simulink model "neuronchainv3"  (Simulink 7.6)
settings: Solver=ode45  StartTime=0.0  StopTime=10.0  RelTol=1e-3
values from neighbouring files (symbols this model uses):
  alpha = 0.8    [excneuroninit.m]
  beta = 0.05    [excneuroninit.m]
  sigslopef = 1    [excneuroninit.m]
  sigslopei = 3    [excneuroninit.m]
  tau_s = 5    [excneuroninit.m]
libraries: simulink x480, neuronpoolibv3 x3
(part 10 of 17)

== system neuronchainv3/Hebbcon2p2/32/h(ui) ==
  x : Inport
  Constant : Constant  Value=offset
  Constant1 : Constant  Value=slope
  Constant2 : Constant
  Gain : Gain  Gain=-1  SaturateOnIntegerOverflow=on  OutDataTypeStr=Inherit: Same as input  ParamDataTypeStr=Inherit: Same as input
  Math Function : Math  SaturateOnIntegerOverflow=on
  Math Function1 : Math  Operator=reciprocal  SaturateOnIntegerOverflow=on
  Model Info : simulink/Model-Wide Utilities/Model Info  SystemSampleTime=-1  InitialBlockCM=None  BlockCM=None  Frame=on  DisplayStringWithTags=|  HorizontalTextAlignment=Center  LeftAlignmentValue=0.5  SourceBlockDiagram=excneuronv3  TagMaxNumber=20
      | Model Info
      | %<Creator> Han, Cheol
  Product : Product  SaturateOnIntegerOverflow=on  OutDataTypeStr=Inherit: Same as first input
  Sum : Sum  Inputs=+-  SaturateOnIntegerOverflow=on
  Sum1 : Sum  SaturateOnIntegerOverflow=on
  y : Outport  InitialOutput=0
  wires:
  x/1 -> Sum/1
  Constant/1 -> Sum/2
  Sum/1 -> Product/1
  Constant1/1 -> Product/2
  Product/1 -> Gain/1
  Gain/1 -> Math Function/1
  Math Function/1 -> Sum1/1
  Constant2/1 -> Sum1/2
  Sum1/1 -> Math Function1/1
  Math Function1/1 -> y/1

== system neuronchainv3/Hebbcon2p2/33/f(ui) ==
  x : Inport
  Constant : Constant  Value=offset
  Constant1 : Constant  Value=slope
  Constant2 : Constant
  Gain : Gain  Gain=-1  SaturateOnIntegerOverflow=on  OutDataTypeStr=Inherit: Same as input  ParamDataTypeStr=Inherit: Same as input
  Math Function : Math  SaturateOnIntegerOverflow=on
  Math Function1 : Math  Operator=reciprocal  SaturateOnIntegerOverflow=on
  Model Info : simulink/Model-Wide Utilities/Model Info  SystemSampleTime=-1  InitialBlockCM=None  BlockCM=None  Frame=on  DisplayStringWithTags=|  HorizontalTextAlignment=Center  LeftAlignmentValue=0.5  SourceBlockDiagram=excneuronv3  TagMaxNumber=20
      | Model Info
      | %<Creator> Han, Cheol
  Product : Product  SaturateOnIntegerOverflow=on  OutDataTypeStr=Inherit: Same as first input
  Sum : Sum  Inputs=+-  SaturateOnIntegerOverflow=on
  Sum1 : Sum  SaturateOnIntegerOverflow=on
  y : Outport  InitialOutput=0
  wires:
  x/1 -> Sum/1
  Constant/1 -> Sum/2
  Sum/1 -> Product/1
  Constant1/1 -> Product/2
  Product/1 -> Gain/1
  Gain/1 -> Math Function/1
  Math Function/1 -> Sum1/1
  Constant2/1 -> Sum1/2
  Sum1/1 -> Math Function1/1
  Math Function1/1 -> y/1

== system neuronchainv3/Hebbcon2p2/33/f(uj) ==
  x : Inport
  Constant : Constant  Value=offset
  Constant1 : Constant  Value=slope
  Constant2 : Constant
  Gain : Gain  Gain=-1  SaturateOnIntegerOverflow=on  OutDataTypeStr=Inherit: Same as input  ParamDataTypeStr=Inherit: Same as input
  Math Function : Math  SaturateOnIntegerOverflow=on
  Math Function1 : Math  Operator=reciprocal  SaturateOnIntegerOverflow=on
  Model Info : simulink/Model-Wide Utilities/Model Info  SystemSampleTime=-1  InitialBlockCM=None  BlockCM=None  Frame=on  DisplayStringWithTags=|  HorizontalTextAlignment=Center  LeftAlignmentValue=0.5  SourceBlockDiagram=excneuronv3  TagMaxNumber=20
      | Model Info
      | %<Creator> Han, Cheol
  Product : Product  SaturateOnIntegerOverflow=on  OutDataTypeStr=Inherit: Same as first input
  Sum : Sum  Inputs=+-  SaturateOnIntegerOverflow=on
  Sum1 : Sum  SaturateOnIntegerOverflow=on
  y : Outport  InitialOutput=0
  wires:
  x/1 -> Sum/1
  Constant/1 -> Sum/2
  Sum/1 -> Product/1
  Constant1/1 -> Product/2
  Product/1 -> Gain/1
  Gain/1 -> Math Function/1
  Math Function/1 -> Sum1/1
  Constant2/1 -> Sum1/2
  Sum1/1 -> Math Function1/1
  Math Function1/1 -> y/1

== system neuronchainv3/Hebbcon2p2/33/h(ui) ==
  x : Inport
  Constant : Constant  Value=offset
  Constant1 : Constant  Value=slope
  Constant2 : Constant
  Gain : Gain  Gain=-1  SaturateOnIntegerOverflow=on  OutDataTypeStr=Inherit: Same as input  ParamDataTypeStr=Inherit: Same as input
  Math Function : Math  SaturateOnIntegerOverflow=on
  Math Function1 : Math  Operator=reciprocal  SaturateOnIntegerOverflow=on
  Model Info : simulink/Model-Wide Utilities/Model Info  SystemSampleTime=-1  InitialBlockCM=None  BlockCM=None  Frame=on  DisplayStringWithTags=|  HorizontalTextAlignment=Center  LeftAlignmentValue=0.5  SourceBlockDiagram=excneuronv3  TagMaxNumber=20
      | Model Info
      | %<Creator> Han, Cheol
  Product : Product  SaturateOnIntegerOverflow=on  OutDataTypeStr=Inherit: Same as first input
  Sum : Sum  Inputs=+-  SaturateOnIntegerOverflow=on
  Sum1 : Sum  SaturateOnIntegerOverflow=on
  y : Outport  InitialOutput=0
  wires:
  x/1 -> Sum/1
  Constant/1 -> Sum/2
  Sum/1 -> Product/1
  Constant1/1 -> Product/2
  Product/1 -> Gain/1
  Gain/1 -> Math Function/1
  Math Function/1 -> Sum1/1
  Constant2/1 -> Sum1/2
  Sum1/1 -> Math Function1/1
  Math Function1/1 -> y/1

== system neuronchainv3/Hebbcon2p2/34/f(ui) ==
  x : Inport
  Constant : Constant  Value=offset
  Constant1 : Constant  Value=slope
  Constant2 : Constant
  Gain : Gain  Gain=-1  SaturateOnIntegerOverflow=on  OutDataTypeStr=Inherit: Same as input  ParamDataTypeStr=Inherit: Same as input
  Math Function : Math  SaturateOnIntegerOverflow=on
  Math Function1 : Math  Operator=reciprocal  SaturateOnIntegerOverflow=on
  Model Info : simulink/Model-Wide Utilities/Model Info  SystemSampleTime=-1  InitialBlockCM=None  BlockCM=None  Frame=on  DisplayStringWithTags=|  HorizontalTextAlignment=Center  LeftAlignmentValue=0.5  SourceBlockDiagram=excneuronv3  TagMaxNumber=20
      | Model Info
      | %<Creator> Han, Cheol
  Product : Product  SaturateOnIntegerOverflow=on  OutDataTypeStr=Inherit: Same as first input
  Sum : Sum  Inputs=+-  SaturateOnIntegerOverflow=on
  Sum1 : Sum  SaturateOnIntegerOverflow=on
  y : Outport  InitialOutput=0
  wires:
  x/1 -> Sum/1
  Constant/1 -> Sum/2
  Sum/1 -> Product/1
  Constant1/1 -> Product/2
  Product/1 -> Gain/1
  Gain/1 -> Math Function/1
  Math Function/1 -> Sum1/1
  Constant2/1 -> Sum1/2
  Sum1/1 -> Math Function1/1
  Math Function1/1 -> y/1

== system neuronchainv3/Hebbcon2p2/34/f(uj) ==
  x : Inport
  Constant : Constant  Value=offset
  Constant1 : Constant  Value=slope
  Constant2 : Constant
  Gain : Gain  Gain=-1  SaturateOnIntegerOverflow=on  OutDataTypeStr=Inherit: Same as input  ParamDataTypeStr=Inherit: Same as input
  Math Function : Math  SaturateOnIntegerOverflow=on
  Math Function1 : Math  Operator=reciprocal  SaturateOnIntegerOverflow=on
  Model Info : simulink/Model-Wide Utilities/Model Info  SystemSampleTime=-1  InitialBlockCM=None  BlockCM=None  Frame=on  DisplayStringWithTags=|  HorizontalTextAlignment=Center  LeftAlignmentValue=0.5  SourceBlockDiagram=excneuronv3  TagMaxNumber=20
      | Model Info
      | %<Creator> Han, Cheol
  Product : Product  SaturateOnIntegerOverflow=on  OutDataTypeStr=Inherit: Same as first input
  Sum : Sum  Inputs=+-  SaturateOnIntegerOverflow=on
  Sum1 : Sum  SaturateOnIntegerOverflow=on
  y : Outport  InitialOutput=0
  wires:
  x/1 -> Sum/1
  Constant/1 -> Sum/2
  Sum/1 -> Product/1
  Constant1/1 -> Product/2
  Product/1 -> Gain/1
  Gain/1 -> Math Function/1
  Math Function/1 -> Sum1/1
  Constant2/1 -> Sum1/2
  Sum1/1 -> Math Function1/1
  Math Function1/1 -> y/1

== system neuronchainv3/Hebbcon2p2/34/h(ui) ==
  x : Inport
  Constant : Constant  Value=offset
  Constant1 : Constant  Value=slope
  Constant2 : Constant
  Gain : Gain  Gain=-1  SaturateOnIntegerOverflow=on  OutDataTypeStr=Inherit: Same as input  ParamDataTypeStr=Inherit: Same as input
  Math Function : Math  SaturateOnIntegerOverflow=on
  Math Function1 : Math  Operator=reciprocal  SaturateOnIntegerOverflow=on
  Model Info : simulink/Model-Wide Utilities/Model Info  SystemSampleTime=-1  InitialBlockCM=None  BlockCM=None  Frame=on  DisplayStringWithTags=|  HorizontalTextAlignment=Center  LeftAlignmentValue=0.5  SourceBlockDiagram=excneuronv3  TagMaxNumber=20
      | Model Info
      | %<Creator> Han, Cheol
  Product : Product  SaturateOnIntegerOverflow=on  OutDataTypeStr=Inherit: Same as first input
  Sum : Sum  Inputs=+-  SaturateOnIntegerOverflow=on
  Sum1 : Sum  SaturateOnIntegerOverflow=on
  y : Outport  InitialOutput=0
  wires:
  x/1 -> Sum/1
  Constant/1 -> Sum/2
  Sum/1 -> Product/1
  Constant1/1 -> Product/2
  Product/1 -> Gain/1
  Gain/1 -> Math Function/1
  Math Function/1 -> Sum1/1
  Constant2/1 -> Sum1/2
  Sum1/1 -> Math Function1/1
  Math Function1/1 -> y/1

== system neuronchainv3/Hebbcon2p2/35/f(ui) ==
  x : Inport
  Constant : Constant  Value=offset
  Constant1 : Constant  Value=slope
  Constant2 : Constant
  Gain : Gain  Gain=-1  SaturateOnIntegerOverflow=on  OutDataTypeStr=Inherit: Same as input  ParamDataTypeStr=Inherit: Same as input
  Math Function : Math  SaturateOnIntegerOverflow=on
  Math Function1 : Math  Operator=reciprocal  SaturateOnIntegerOverflow=on
  Model Info : simulink/Model-Wide Utilities/Model Info  SystemSampleTime=-1  InitialBlockCM=None  BlockCM=None  Frame=on  DisplayStringWithTags=|  HorizontalTextAlignment=Center  LeftAlignmentValue=0.5  SourceBlockDiagram=excneuronv3  TagMaxNumber=20
      | Model Info
      | %<Creator> Han, Cheol
  Product : Product  SaturateOnIntegerOverflow=on  OutDataTypeStr=Inherit: Same as first input
  Sum : Sum  Inputs=+-  SaturateOnIntegerOverflow=on
  Sum1 : Sum  SaturateOnIntegerOverflow=on
  y : Outport  InitialOutput=0
  wires:
  x/1 -> Sum/1
  Constant/1 -> Sum/2
  Sum/1 -> Product/1
  Constant1/1 -> Product/2
  Product/1 -> Gain/1
  Gain/1 -> Math Function/1
  Math Function/1 -> Sum1/1
  Constant2/1 -> Sum1/2
  Sum1/1 -> Math Function1/1
  Math Function1/1 -> y/1

== system neuronchainv3/Hebbcon2p2/35/f(uj) ==
  x : Inport
  Constant : Constant  Value=offset
  Constant1 : Constant  Value=slope
  Constant2 : Constant
  Gain : Gain  Gain=-1  SaturateOnIntegerOverflow=on  OutDataTypeStr=Inherit: Same as input  ParamDataTypeStr=Inherit: Same as input
  Math Function : Math  SaturateOnIntegerOverflow=on
  Math Function1 : Math  Operator=reciprocal  SaturateOnIntegerOverflow=on
  Model Info : simulink/Model-Wide Utilities/Model Info  SystemSampleTime=-1  InitialBlockCM=None  BlockCM=None  Frame=on  DisplayStringWithTags=|  HorizontalTextAlignment=Center  LeftAlignmentValue=0.5  SourceBlockDiagram=excneuronv3  TagMaxNumber=20
      | Model Info
      | %<Creator> Han, Cheol
  Product : Product  SaturateOnIntegerOverflow=on  OutDataTypeStr=Inherit: Same as first input
  Sum : Sum  Inputs=+-  SaturateOnIntegerOverflow=on
  Sum1 : Sum  SaturateOnIntegerOverflow=on
  y : Outport  InitialOutput=0
  wires:
  x/1 -> Sum/1
  Constant/1 -> Sum/2
  Sum/1 -> Product/1
  Constant1/1 -> Product/2
  Product/1 -> Gain/1
  Gain/1 -> Math Function/1
  Math Function/1 -> Sum1/1
  Constant2/1 -> Sum1/2
  Sum1/1 -> Math Function1/1
  Math Function1/1 -> y/1

== system neuronchainv3/Hebbcon2p2/35/h(ui) ==
  x : Inport
  Constant : Constant  Value=offset
  Constant1 : Constant  Value=slope
  Constant2 : Constant
  Gain : Gain  Gain=-1  SaturateOnIntegerOverflow=on  OutDataTypeStr=Inherit: Same as input  ParamDataTypeStr=Inherit: Same as input
  Math Function : Math  SaturateOnIntegerOverflow=on
  Math Function1 : Math  Operator=reciprocal  SaturateOnIntegerOverflow=on
  Model Info : simulink/Model-Wide Utilities/Model Info  SystemSampleTime=-1  InitialBlockCM=None  BlockCM=None  Frame=on  DisplayStringWithTags=|  HorizontalTextAlignment=Center  LeftAlignmentValue=0.5  SourceBlockDiagram=excneuronv3  TagMaxNumber=20
      | Model Info
      | %<Creator> Han, Cheol
  Product : Product  SaturateOnIntegerOverflow=on  OutDataTypeStr=Inherit: Same as first input
  Sum : Sum  Inputs=+-  SaturateOnIntegerOverflow=on
  Sum1 : Sum  SaturateOnIntegerOverflow=on
  y : Outport  InitialOutput=0
  wires:
  x/1 -> Sum/1
  Constant/1 -> Sum/2
  Sum/1 -> Product/1
  Constant1/1 -> Product/2
  Product/1 -> Gain/1
  Gain/1 -> Math Function/1
  Math Function/1 -> Sum1/1
  Constant2/1 -> Sum1/2
  Sum1/1 -> Math Function1/1
  Math Function1/1 -> y/1

== system neuronchainv3/Hebbcon2p2/4/f(ui) ==
  x : Inport
  Constant : Constant  Value=offset
  Constant1 : Constant  Value=slope
  Constant2 : Constant
  Gain : Gain  Gain=-1  SaturateOnIntegerOverflow=on  OutDataTypeStr=Inherit: Same as input  ParamDataTypeStr=Inherit: Same as input
  Math Function : Math  SaturateOnIntegerOverflow=on
  Math Function1 : Math  Operator=reciprocal  SaturateOnIntegerOverflow=on
  Model Info : simulink/Model-Wide Utilities/Model Info  SystemSampleTime=-1  InitialBlockCM=None  BlockCM=None  Frame=on  DisplayStringWithTags=|  HorizontalTextAlignment=Center  LeftAlignmentValue=0.5  SourceBlockDiagram=excneuronv3  TagMaxNumber=20
      | Model Info
      | %<Creator> Han, Cheol
  Product : Product  SaturateOnIntegerOverflow=on  OutDataTypeStr=Inherit: Same as first input
  Sum : Sum  Inputs=+-  SaturateOnIntegerOverflow=on
  Sum1 : Sum  SaturateOnIntegerOverflow=on
  y : Outport  InitialOutput=0
  wires:
  x/1 -> Sum/1
  Constant/1 -> Sum/2
  Sum/1 -> Product/1
  Constant1/1 -> Product/2
  Product/1 -> Gain/1
  Gain/1 -> Math Function/1
  Math Function/1 -> Sum1/1
  Constant2/1 -> Sum1/2
  Sum1/1 -> Math Function1/1
  Math Function1/1 -> y/1

== system neuronchainv3/Hebbcon2p2/4/f(uj) ==
  x : Inport
  Constant : Constant  Value=offset
  Constant1 : Constant  Value=slope
  Constant2 : Constant
  Gain : Gain  Gain=-1  SaturateOnIntegerOverflow=on  OutDataTypeStr=Inherit: Same as input  ParamDataTypeStr=Inherit: Same as input
  Math Function : Math  SaturateOnIntegerOverflow=on
  Math Function1 : Math  Operator=reciprocal  SaturateOnIntegerOverflow=on
  Model Info : simulink/Model-Wide Utilities/Model Info  SystemSampleTime=-1  InitialBlockCM=None  BlockCM=None  Frame=on  DisplayStringWithTags=|  HorizontalTextAlignment=Center  LeftAlignmentValue=0.5  SourceBlockDiagram=excneuronv3  TagMaxNumber=20
      | Model Info
      | %<Creator> Han, Cheol
  Product : Product  SaturateOnIntegerOverflow=on  OutDataTypeStr=Inherit: Same as first input
  Sum : Sum  Inputs=+-  SaturateOnIntegerOverflow=on
  Sum1 : Sum  SaturateOnIntegerOverflow=on
  y : Outport  InitialOutput=0
  wires:
  x/1 -> Sum/1
  Constant/1 -> Sum/2
  Sum/1 -> Product/1
  Constant1/1 -> Product/2
  Product/1 -> Gain/1
  Gain/1 -> Math Function/1
  Math Function/1 -> Sum1/1
  Constant2/1 -> Sum1/2
  Sum1/1 -> Math Function1/1
  Math Function1/1 -> y/1

== system neuronchainv3/Hebbcon2p2/4/h(ui) ==
  x : Inport
  Constant : Constant  Value=offset
  Constant1 : Constant  Value=slope
  Constant2 : Constant
  Gain : Gain  Gain=-1  SaturateOnIntegerOverflow=on  OutDataTypeStr=Inherit: Same as input  ParamDataTypeStr=Inherit: Same as input
  Math Function : Math  SaturateOnIntegerOverflow=on
  Math Function1 : Math  Operator=reciprocal  SaturateOnIntegerOverflow=on
  Model Info : simulink/Model-Wide Utilities/Model Info  SystemSampleTime=-1  InitialBlockCM=None  BlockCM=None  Frame=on  DisplayStringWithTags=|  HorizontalTextAlignment=Center  LeftAlignmentValue=0.5  SourceBlockDiagram=excneuronv3  TagMaxNumber=20
      | Model Info
      | %<Creator> Han, Cheol
  Product : Product  SaturateOnIntegerOverflow=on  OutDataTypeStr=Inherit: Same as first input
  Sum : Sum  Inputs=+-  SaturateOnIntegerOverflow=on
  Sum1 : Sum  SaturateOnIntegerOverflow=on
  y : Outport  InitialOutput=0
  wires:
  x/1 -> Sum/1
  Constant/1 -> Sum/2
  Sum/1 -> Product/1
  Constant1/1 -> Product/2
  Product/1 -> Gain/1
  Gain/1 -> Math Function/1
  Math Function/1 -> Sum1/1
  Constant2/1 -> Sum1/2
  Sum1/1 -> Math Function1/1
  Math Function1/1 -> y/1

== system neuronchainv3/Hebbcon2p2/41/f(ui) ==
  x : Inport
  Constant : Constant  Value=offset
  Constant1 : Constant  Value=slope
  Constant2 : Constant
  Gain : Gain  Gain=-1  SaturateOnIntegerOverflow=on  OutDataTypeStr=Inherit: Same as input  ParamDataTypeStr=Inherit: Same as input
  Math Function : Math  SaturateOnIntegerOverflow=on
  Math Function1 : Math  Operator=reciprocal  SaturateOnIntegerOverflow=on
  Model Info : simulink/Model-Wide Utilities/Model Info  SystemSampleTime=-1  InitialBlockCM=None  BlockCM=None  Frame=on  DisplayStringWithTags=|  HorizontalTextAlignment=Center  LeftAlignmentValue=0.5  SourceBlockDiagram=excneuronv3  TagMaxNumber=20
      | Model Info
      | %<Creator> Han, Cheol
  Product : Product  SaturateOnIntegerOverflow=on  OutDataTypeStr=Inherit: Same as first input
  Sum : Sum  Inputs=+-  SaturateOnIntegerOverflow=on
  Sum1 : Sum  SaturateOnIntegerOverflow=on
  y : Outport  InitialOutput=0
  wires:
  x/1 -> Sum/1
  Constant/1 -> Sum/2
  Sum/1 -> Product/1
  Constant1/1 -> Product/2
  Product/1 -> Gain/1
  Gain/1 -> Math Function/1
  Math Function/1 -> Sum1/1
  Constant2/1 -> Sum1/2
  Sum1/1 -> Math Function1/1
  Math Function1/1 -> y/1

== system neuronchainv3/Hebbcon2p2/41/f(uj) ==
  x : Inport
  Constant : Constant  Value=offset
  Constant1 : Constant  Value=slope
  Constant2 : Constant
  Gain : Gain  Gain=-1  SaturateOnIntegerOverflow=on  OutDataTypeStr=Inherit: Same as input  ParamDataTypeStr=Inherit: Same as input
  Math Function : Math  SaturateOnIntegerOverflow=on
  Math Function1 : Math  Operator=reciprocal  SaturateOnIntegerOverflow=on
  Model Info : simulink/Model-Wide Utilities/Model Info  SystemSampleTime=-1  InitialBlockCM=None  BlockCM=None  Frame=on  DisplayStringWithTags=|  HorizontalTextAlignment=Center  LeftAlignmentValue=0.5  SourceBlockDiagram=excneuronv3  TagMaxNumber=20
      | Model Info
      | %<Creator> Han, Cheol
  Product : Product  SaturateOnIntegerOverflow=on  OutDataTypeStr=Inherit: Same as first input
  Sum : Sum  Inputs=+-  SaturateOnIntegerOverflow=on
  Sum1 : Sum  SaturateOnIntegerOverflow=on
  y : Outport  InitialOutput=0
  wires:
  x/1 -> Sum/1
  Constant/1 -> Sum/2
  Sum/1 -> Product/1
  Constant1/1 -> Product/2
  Product/1 -> Gain/1
  Gain/1 -> Math Function/1
  Math Function/1 -> Sum1/1
  Constant2/1 -> Sum1/2
  Sum1/1 -> Math Function1/1
  Math Function1/1 -> y/1

== system neuronchainv3/Hebbcon2p2/41/h(ui) ==
  x : Inport
  Constant : Constant  Value=offset
  Constant1 : Constant  Value=slope
  Constant2 : Constant
  Gain : Gain  Gain=-1  SaturateOnIntegerOverflow=on  OutDataTypeStr=Inherit: Same as input  ParamDataTypeStr=Inherit: Same as input
  Math Function : Math  SaturateOnIntegerOverflow=on
  Math Function1 : Math  Operator=reciprocal  SaturateOnIntegerOverflow=on
  Model Info : simulink/Model-Wide Utilities/Model Info  SystemSampleTime=-1  InitialBlockCM=None  BlockCM=None  Frame=on  DisplayStringWithTags=|  HorizontalTextAlignment=Center  LeftAlignmentValue=0.5  SourceBlockDiagram=excneuronv3  TagMaxNumber=20
      | Model Info
      | %<Creator> Han, Cheol
  Product : Product  SaturateOnIntegerOverflow=on  OutDataTypeStr=Inherit: Same as first input
  Sum : Sum  Inputs=+-  SaturateOnIntegerOverflow=on
  Sum1 : Sum  SaturateOnIntegerOverflow=on
  y : Outport  InitialOutput=0
  wires:
  x/1 -> Sum/1
  Constant/1 -> Sum/2
  Sum/1 -> Product/1
  Constant1/1 -> Product/2
  Product/1 -> Gain/1
  Gain/1 -> Math Function/1
  Math Function/1 -> Sum1/1
  Constant2/1 -> Sum1/2
  Sum1/1 -> Math Function1/1
  Math Function1/1 -> y/1

== system neuronchainv3/Hebbcon2p2/42/f(ui) ==
  x : Inport
  Constant : Constant  Value=offset
  Constant1 : Constant  Value=slope
  Constant2 : Constant
  Gain : Gain  Gain=-1  SaturateOnIntegerOverflow=on  OutDataTypeStr=Inherit: Same as input  ParamDataTypeStr=Inherit: Same as input
  Math Function : Math  SaturateOnIntegerOverflow=on
  Math Function1 : Math  Operator=reciprocal  SaturateOnIntegerOverflow=on
  Model Info : simulink/Model-Wide Utilities/Model Info  SystemSampleTime=-1  InitialBlockCM=None  BlockCM=None  Frame=on  DisplayStringWithTags=|  HorizontalTextAlignment=Center  LeftAlignmentValue=0.5  SourceBlockDiagram=excneuronv3  TagMaxNumber=20
      | Model Info
      | %<Creator> Han, Cheol
  Product : Product  SaturateOnIntegerOverflow=on  OutDataTypeStr=Inherit: Same as first input
  Sum : Sum  Inputs=+-  SaturateOnIntegerOverflow=on
  Sum1 : Sum  SaturateOnIntegerOverflow=on
  y : Outport  InitialOutput=0
  wires:
  x/1 -> Sum/1
  Constant/1 -> Sum/2
  Sum/1 -> Product/1
  Constant1/1 -> Product/2
  Product/1 -> Gain/1
  Gain/1 -> Math Function/1
  Math Function/1 -> Sum1/1
  Constant2/1 -> Sum1/2
  Sum1/1 -> Math Function1/1
  Math Function1/1 -> y/1

== system neuronchainv3/Hebbcon2p2/42/f(uj) ==
  x : Inport
  Constant : Constant  Value=offset
  Constant1 : Constant  Value=slope
  Constant2 : Constant
  Gain : Gain  Gain=-1  SaturateOnIntegerOverflow=on  OutDataTypeStr=Inherit: Same as input  ParamDataTypeStr=Inherit: Same as input
  Math Function : Math  SaturateOnIntegerOverflow=on
  Math Function1 : Math  Operator=reciprocal  SaturateOnIntegerOverflow=on
  Model Info : simulink/Model-Wide Utilities/Model Info  SystemSampleTime=-1  InitialBlockCM=None  BlockCM=None  Frame=on  DisplayStringWithTags=|  HorizontalTextAlignment=Center  LeftAlignmentValue=0.5  SourceBlockDiagram=excneuronv3  TagMaxNumber=20
      | Model Info
      | %<Creator> Han, Cheol
  Product : Product  SaturateOnIntegerOverflow=on  OutDataTypeStr=Inherit: Same as first input
  Sum : Sum  Inputs=+-  SaturateOnIntegerOverflow=on
  Sum1 : Sum  SaturateOnIntegerOverflow=on
  y : Outport  InitialOutput=0
  wires:
  x/1 -> Sum/1
  Constant/1 -> Sum/2
  Sum/1 -> Product/1
  Constant1/1 -> Product/2
  Product/1 -> Gain/1
  Gain/1 -> Math Function/1
  Math Function/1 -> Sum1/1
  Constant2/1 -> Sum1/2
  Sum1/1 -> Math Function1/1
  Math Function1/1 -> y/1

== system neuronchainv3/Hebbcon2p2/42/h(ui) ==
  x : Inport
  Constant : Constant  Value=offset
  Constant1 : Constant  Value=slope
  Constant2 : Constant
  Gain : Gain  Gain=-1  SaturateOnIntegerOverflow=on  OutDataTypeStr=Inherit: Same as input  ParamDataTypeStr=Inherit: Same as input
  Math Function : Math  SaturateOnIntegerOverflow=on
  Math Function1 : Math  Operator=reciprocal  SaturateOnIntegerOverflow=on
  Model Info : simulink/Model-Wide Utilities/Model Info  SystemSampleTime=-1  InitialBlockCM=None  BlockCM=None  Frame=on  DisplayStringWithTags=|  HorizontalTextAlignment=Center  LeftAlignmentValue=0.5  SourceBlockDiagram=excneuronv3  TagMaxNumber=20
      | Model Info
      | %<Creator> Han, Cheol
  Product : Product  SaturateOnIntegerOverflow=on  OutDataTypeStr=Inherit: Same as first input
  Sum : Sum  Inputs=+-  SaturateOnIntegerOverflow=on
  Sum1 : Sum  SaturateOnIntegerOverflow=on
  y : Outport  InitialOutput=0
  wires:
  x/1 -> Sum/1
  Constant/1 -> Sum/2
  Sum/1 -> Product/1
  Constant1/1 -> Product/2
  Product/1 -> Gain/1
  Gain/1 -> Math Function/1
  Math Function/1 -> Sum1/1
  Constant2/1 -> Sum1/2
  Sum1/1 -> Math Function1/1
  Math Function1/1 -> y/1

== system neuronchainv3/Hebbcon2p2/43/f(ui) ==
  x : Inport
  Constant : Constant  Value=offset
  Constant1 : Constant  Value=slope
  Constant2 : Constant
  Gain : Gain  Gain=-1  SaturateOnIntegerOverflow=on  OutDataTypeStr=Inherit: Same as input  ParamDataTypeStr=Inherit: Same as input
  Math Function : Math  SaturateOnIntegerOverflow=on
  Math Function1 : Math  Operator=reciprocal  SaturateOnIntegerOverflow=on
  Model Info : simulink/Model-Wide Utilities/Model Info  SystemSampleTime=-1  InitialBlockCM=None  BlockCM=None  Frame=on  DisplayStringWithTags=|  HorizontalTextAlignment=Center  LeftAlignmentValue=0.5  SourceBlockDiagram=excneuronv3  TagMaxNumber=20
      | Model Info
      | %<Creator> Han, Cheol
  Product : Product  SaturateOnIntegerOverflow=on  OutDataTypeStr=Inherit: Same as first input
  Sum : Sum  Inputs=+-  SaturateOnIntegerOverflow=on
  Sum1 : Sum  SaturateOnIntegerOverflow=on
  y : Outport  InitialOutput=0
  wires:
  x/1 -> Sum/1
  Constant/1 -> Sum/2
  Sum/1 -> Product/1
  Constant1/1 -> Product/2
  Product/1 -> Gain/1
  Gain/1 -> Math Function/1
  Math Function/1 -> Sum1/1
  Constant2/1 -> Sum1/2
  Sum1/1 -> Math Function1/1
  Math Function1/1 -> y/1

== system neuronchainv3/Hebbcon2p2/43/f(uj) ==
  x : Inport
  Constant : Constant  Value=offset
  Constant1 : Constant  Value=slope
  Constant2 : Constant
  Gain : Gain  Gain=-1  SaturateOnIntegerOverflow=on  OutDataTypeStr=Inherit: Same as input  ParamDataTypeStr=Inherit: Same as input
  Math Function : Math  SaturateOnIntegerOverflow=on
  Math Function1 : Math  Operator=reciprocal  SaturateOnIntegerOverflow=on
  Model Info : simulink/Model-Wide Utilities/Model Info  SystemSampleTime=-1  InitialBlockCM=None  BlockCM=None  Frame=on  DisplayStringWithTags=|  HorizontalTextAlignment=Center  LeftAlignmentValue=0.5  SourceBlockDiagram=excneuronv3  TagMaxNumber=20
      | Model Info
      | %<Creator> Han, Cheol
  Product : Product  SaturateOnIntegerOverflow=on  OutDataTypeStr=Inherit: Same as first input
  Sum : Sum  Inputs=+-  SaturateOnIntegerOverflow=on
  Sum1 : Sum  SaturateOnIntegerOverflow=on
  y : Outport  InitialOutput=0
  wires:
  x/1 -> Sum/1
  Constant/1 -> Sum/2
  Sum/1 -> Product/1
  Constant1/1 -> Product/2
  Product/1 -> Gain/1
  Gain/1 -> Math Function/1
  Math Function/1 -> Sum1/1
  Constant2/1 -> Sum1/2
  Sum1/1 -> Math Function1/1
  Math Function1/1 -> y/1

== system neuronchainv3/Hebbcon2p2/43/h(ui) ==
  x : Inport
  Constant : Constant  Value=offset
  Constant1 : Constant  Value=slope
  Constant2 : Constant
  Gain : Gain  Gain=-1  SaturateOnIntegerOverflow=on  OutDataTypeStr=Inherit: Same as input  ParamDataTypeStr=Inherit: Same as input
  Math Function : Math  SaturateOnIntegerOverflow=on
  Math Function1 : Math  Operator=reciprocal  SaturateOnIntegerOverflow=on
  Model Info : simulink/Model-Wide Utilities/Model Info  SystemSampleTime=-1  InitialBlockCM=None  BlockCM=None  Frame=on  DisplayStringWithTags=|  HorizontalTextAlignment=Center  LeftAlignmentValue=0.5  SourceBlockDiagram=excneuronv3  TagMaxNumber=20
      | Model Info
      | %<Creator> Han, Cheol
  Product : Product  SaturateOnIntegerOverflow=on  OutDataTypeStr=Inherit: Same as first input
  Sum : Sum  Inputs=+-  SaturateOnIntegerOverflow=on
  Sum1 : Sum  SaturateOnIntegerOverflow=on
  y : Outport  InitialOutput=0
  wires:
  x/1 -> Sum/1
  Constant/1 -> Sum/2
  Sum/1 -> Product/1
  Constant1/1 -> Product/2
  Product/1 -> Gain/1
  Gain/1 -> Math Function/1
  Math Function/1 -> Sum1/1
  Constant2/1 -> Sum1/2
  Sum1/1 -> Math Function1/1
  Math Function1/1 -> y/1

== system neuronchainv3/Hebbcon2p2/44/f(ui) ==
  x : Inport
  Constant : Constant  Value=offset
  Constant1 : Constant  Value=slope
  Constant2 : Constant
  Gain : Gain  Gain=-1  SaturateOnIntegerOverflow=on  OutDataTypeStr=Inherit: Same as input  ParamDataTypeStr=Inherit: Same as input
  Math Function : Math  SaturateOnIntegerOverflow=on
  Math Function1 : Math  Operator=reciprocal  SaturateOnIntegerOverflow=on
  Model Info : simulink/Model-Wide Utilities/Model Info  SystemSampleTime=-1  InitialBlockCM=None  BlockCM=None  Frame=on  DisplayStringWithTags=|  HorizontalTextAlignment=Center  LeftAlignmentValue=0.5  SourceBlockDiagram=excneuronv3  TagMaxNumber=20
      | Model Info
      | %<Creator> Han, Cheol
  Product : Product  SaturateOnIntegerOverflow=on  OutDataTypeStr=Inherit: Same as first input
  Sum : Sum  Inputs=+-  SaturateOnIntegerOverflow=on
  Sum1 : Sum  SaturateOnIntegerOverflow=on
  y : Outport  InitialOutput=0
  wires:
  x/1 -> Sum/1
  Constant/1 -> Sum/2
  Sum/1 -> Product/1
  Constant1/1 -> Product/2
  Product/1 -> Gain/1
  Gain/1 -> Math Function/1
  Math Function/1 -> Sum1/1
  Constant2/1 -> Sum1/2
  Sum1/1 -> Math Function1/1
  Math Function1/1 -> y/1

== system neuronchainv3/Hebbcon2p2/44/f(uj) ==
  x : Inport
  Constant : Constant  Value=offset
  Constant1 : Constant  Value=slope
  Constant2 : Constant
  Gain : Gain  Gain=-1  SaturateOnIntegerOverflow=on  OutDataTypeStr=Inherit: Same as input  ParamDataTypeStr=Inherit: Same as input
  Math Function : Math  SaturateOnIntegerOverflow=on
  Math Function1 : Math  Operator=reciprocal  SaturateOnIntegerOverflow=on
  Model Info : simulink/Model-Wide Utilities/Model Info  SystemSampleTime=-1  InitialBlockCM=None  BlockCM=None  Frame=on  DisplayStringWithTags=|  HorizontalTextAlignment=Center  LeftAlignmentValue=0.5  SourceBlockDiagram=excneuronv3  TagMaxNumber=20
      | Model Info
      | %<Creator> Han, Cheol
  Product : Product  SaturateOnIntegerOverflow=on  OutDataTypeStr=Inherit: Same as first input
  Sum : Sum  Inputs=+-  SaturateOnIntegerOverflow=on
  Sum1 : Sum  SaturateOnIntegerOverflow=on
  y : Outport  InitialOutput=0
  wires:
  x/1 -> Sum/1
  Constant/1 -> Sum/2
  Sum/1 -> Product/1
  Constant1/1 -> Product/2
  Product/1 -> Gain/1
  Gain/1 -> Math Function/1
  Math Function/1 -> Sum1/1
  Constant2/1 -> Sum1/2
  Sum1/1 -> Math Function1/1
  Math Function1/1 -> y/1

== system neuronchainv3/Hebbcon2p2/44/h(ui) ==
  x : Inport
  Constant : Constant  Value=offset
  Constant1 : Constant  Value=slope
  Constant2 : Constant
  Gain : Gain  Gain=-1  SaturateOnIntegerOverflow=on  OutDataTypeStr=Inherit: Same as input  ParamDataTypeStr=Inherit: Same as input
  Math Function : Math  SaturateOnIntegerOverflow=on
  Math Function1 : Math  Operator=reciprocal  SaturateOnIntegerOverflow=on
  Model Info : simulink/Model-Wide Utilities/Model Info  SystemSampleTime=-1  InitialBlockCM=None  BlockCM=None  Frame=on  DisplayStringWithTags=|  HorizontalTextAlignment=Center  LeftAlignmentValue=0.5  SourceBlockDiagram=excneuronv3  TagMaxNumber=20
      | Model Info
      | %<Creator> Han, Cheol
  Product : Product  SaturateOnIntegerOverflow=on  OutDataTypeStr=Inherit: Same as first input
  Sum : Sum  Inputs=+-  SaturateOnIntegerOverflow=on
  Sum1 : Sum  SaturateOnIntegerOverflow=on
  y : Outport  InitialOutput=0
  wires:
  x/1 -> Sum/1
  Constant/1 -> Sum/2
  Sum/1 -> Product/1
  Constant1/1 -> Product/2
  Product/1 -> Gain/1
  Gain/1 -> Math Function/1
  Math Function/1 -> Sum1/1
  Constant2/1 -> Sum1/2
  Sum1/1 -> Math Function1/1
  Math Function1/1 -> y/1

== system neuronchainv3/Hebbcon2p2/45/f(ui) ==
  x : Inport
  Constant : Constant  Value=offset
  Constant1 : Constant  Value=slope
  Constant2 : Constant
  Gain : Gain  Gain=-1  SaturateOnIntegerOverflow=on  OutDataTypeStr=Inherit: Same as input  ParamDataTypeStr=Inherit: Same as input
  Math Function : Math  SaturateOnIntegerOverflow=on
  Math Function1 : Math  Operator=reciprocal  SaturateOnIntegerOverflow=on
  Model Info : simulink/Model-Wide Utilities/Model Info  SystemSampleTime=-1  InitialBlockCM=None  BlockCM=None  Frame=on  DisplayStringWithTags=|  HorizontalTextAlignment=Center  LeftAlignmentValue=0.5  SourceBlockDiagram=excneuronv3  TagMaxNumber=20
      | Model Info
      | %<Creator> Han, Cheol
  Product : Product  SaturateOnIntegerOverflow=on  OutDataTypeStr=Inherit: Same as first input
  Sum : Sum  Inputs=+-  SaturateOnIntegerOverflow=on
  Sum1 : Sum  SaturateOnIntegerOverflow=on
  y : Outport  InitialOutput=0
  wires:
  x/1 -> Sum/1
  Constant/1 -> Sum/2
  Sum/1 -> Product/1
  Constant1/1 -> Product/2
  Product/1 -> Gain/1
  Gain/1 -> Math Function/1
  Math Function/1 -> Sum1/1
  Constant2/1 -> Sum1/2
  Sum1/1 -> Math Function1/1
  Math Function1/1 -> y/1

== system neuronchainv3/Hebbcon2p2/45/f(uj) ==
  x : Inport
  Constant : Constant  Value=offset
  Constant1 : Constant  Value=slope
  Constant2 : Constant
  Gain : Gain  Gain=-1  SaturateOnIntegerOverflow=on  OutDataTypeStr=Inherit: Same as input  ParamDataTypeStr=Inherit: Same as input
  Math Function : Math  SaturateOnIntegerOverflow=on
  Math Function1 : Math  Operator=reciprocal  SaturateOnIntegerOverflow=on
  Model Info : simulink/Model-Wide Utilities/Model Info  SystemSampleTime=-1  InitialBlockCM=None  BlockCM=None  Frame=on  DisplayStringWithTags=|  HorizontalTextAlignment=Center  LeftAlignmentValue=0.5  SourceBlockDiagram=excneuronv3  TagMaxNumber=20
      | Model Info
      | %<Creator> Han, Cheol
  Product : Product  SaturateOnIntegerOverflow=on  OutDataTypeStr=Inherit: Same as first input
  Sum : Sum  Inputs=+-  SaturateOnIntegerOverflow=on
  Sum1 : Sum  SaturateOnIntegerOverflow=on
  y : Outport  InitialOutput=0
  wires:
  x/1 -> Sum/1
  Constant/1 -> Sum/2
  Sum/1 -> Product/1
  Constant1/1 -> Product/2
  Product/1 -> Gain/1
  Gain/1 -> Math Function/1
  Math Function/1 -> Sum1/1
  Constant2/1 -> Sum1/2
  Sum1/1 -> Math Function1/1
  Math Function1/1 -> y/1

== system neuronchainv3/Hebbcon2p2/45/h(ui) ==
  x : Inport
  Constant : Constant  Value=offset
  Constant1 : Constant  Value=slope
  Constant2 : Constant
  Gain : Gain  Gain=-1  SaturateOnIntegerOverflow=on  OutDataTypeStr=Inherit: Same as input  ParamDataTypeStr=Inherit: Same as input
  Math Function : Math  SaturateOnIntegerOverflow=on
  Math Function1 : Math  Operator=reciprocal  SaturateOnIntegerOverflow=on
  Model Info : simulink/Model-Wide Utilities/Model Info  SystemSampleTime=-1  InitialBlockCM=None  BlockCM=None  Frame=on  DisplayStringWithTags=|  HorizontalTextAlignment=Center  LeftAlignmentValue=0.5  SourceBlockDiagram=excneuronv3  TagMaxNumber=20
      | Model Info
      | %<Creator> Han, Cheol
  Product : Product  SaturateOnIntegerOverflow=on  OutDataTypeStr=Inherit: Same as first input
  Sum : Sum  Inputs=+-  SaturateOnIntegerOverflow=on
  Sum1 : Sum  SaturateOnIntegerOverflow=on
  y : Outport  InitialOutput=0
  wires:
  x/1 -> Sum/1
  Constant/1 -> Sum/2
  Sum/1 -> Product/1
  Constant1/1 -> Product/2
  Product/1 -> Gain/1
  Gain/1 -> Math Function/1
  Math Function/1 -> Sum1/1
  Constant2/1 -> Sum1/2
  Sum1/1 -> Math Function1/1
  Math Function1/1 -> y/1

== system neuronchainv3/Hebbcon2p2/5/f(ui) ==
  x : Inport
  Constant : Constant  Value=offset
  Constant1 : Constant  Value=slope
  Constant2 : Constant
  Gain : Gain  Gain=-1  SaturateOnIntegerOverflow=on  OutDataTypeStr=Inherit: Same as input  ParamDataTypeStr=Inherit: Same as input
  Math Function : Math  SaturateOnIntegerOverflow=on
  Math Function1 : Math  Operator=reciprocal  SaturateOnIntegerOverflow=on
  Model Info : simulink/Model-Wide Utilities/Model Info  SystemSampleTime=-1  InitialBlockCM=None  BlockCM=None  Frame=on  DisplayStringWithTags=|  HorizontalTextAlignment=Center  LeftAlignmentValue=0.5  SourceBlockDiagram=excneuronv3  TagMaxNumber=20
      | Model Info
      | %<Creator> Han, Cheol
  Product : Product  SaturateOnIntegerOverflow=on  OutDataTypeStr=Inherit: Same as first input
  Sum : Sum  Inputs=+-  SaturateOnIntegerOverflow=on
  Sum1 : Sum  SaturateOnIntegerOverflow=on
  y : Outport  InitialOutput=0
  wires:
  x/1 -> Sum/1
  Constant/1 -> Sum/2
  Sum/1 -> Product/1
  Constant1/1 -> Product/2
  Product/1 -> Gain/1
  Gain/1 -> Math Function/1
  Math Function/1 -> Sum1/1
  Constant2/1 -> Sum1/2
  Sum1/1 -> Math Function1/1
  Math Function1/1 -> y/1

== system neuronchainv3/Hebbcon2p2/5/f(uj) ==
  x : Inport
  Constant : Constant  Value=offset
  Constant1 : Constant  Value=slope
  Constant2 : Constant
  Gain : Gain  Gain=-1  SaturateOnIntegerOverflow=on  OutDataTypeStr=Inherit: Same as input  ParamDataTypeStr=Inherit: Same as input
  Math Function : Math  SaturateOnIntegerOverflow=on
  Math Function1 : Math  Operator=reciprocal  SaturateOnIntegerOverflow=on
  Model Info : simulink/Model-Wide Utilities/Model Info  SystemSampleTime=-1  InitialBlockCM=None  BlockCM=None  Frame=on  DisplayStringWithTags=|  HorizontalTextAlignment=Center  LeftAlignmentValue=0.5  SourceBlockDiagram=excneuronv3  TagMaxNumber=20
      | Model Info
      | %<Creator> Han, Cheol
  Product : Product  SaturateOnIntegerOverflow=on  OutDataTypeStr=Inherit: Same as first input
  Sum : Sum  Inputs=+-  SaturateOnIntegerOverflow=on
  Sum1 : Sum  SaturateOnIntegerOverflow=on
  y : Outport  InitialOutput=0
  wires:
  x/1 -> Sum/1
  Constant/1 -> Sum/2
  Sum/1 -> Product/1
  Constant1/1 -> Product/2
  Product/1 -> Gain/1
  Gain/1 -> Math Function/1
  Math Function/1 -> Sum1/1
  Constant2/1 -> Sum1/2
  Sum1/1 -> Math Function1/1
  Math Function1/1 -> y/1

== system neuronchainv3/Hebbcon2p2/5/h(ui) ==
  x : Inport
  Constant : Constant  Value=offset
  Constant1 : Constant  Value=slope
  Constant2 : Constant
  Gain : Gain  Gain=-1  SaturateOnIntegerOverflow=on  OutDataTypeStr=Inherit: Same as input  ParamDataTypeStr=Inherit: Same as input
  Math Function : Math  SaturateOnIntegerOverflow=on
  Math Function1 : Math  Operator=reciprocal  SaturateOnIntegerOverflow=on
  Model Info : simulink/Model-Wide Utilities/Model Info  SystemSampleTime=-1  InitialBlockCM=None  BlockCM=None  Frame=on  DisplayStringWithTags=|  HorizontalTextAlignment=Center  LeftAlignmentValue=0.5  SourceBlockDiagram=excneuronv3  TagMaxNumber=20
      | Model Info
      | %<Creator> Han, Cheol
  Product : Product  SaturateOnIntegerOverflow=on  OutDataTypeStr=Inherit: Same as first input
  Sum : Sum  Inputs=+-  SaturateOnIntegerOverflow=on
  Sum1 : Sum  SaturateOnIntegerOverflow=on
  y : Outport  InitialOutput=0
  wires:
  x/1 -> Sum/1
  Constant/1 -> Sum/2
  Sum/1 -> Product/1
  Constant1/1 -> Product/2
  Product/1 -> Gain/1
  Gain/1 -> Math Function/1
  Math Function/1 -> Sum1/1
  Constant2/1 -> Sum1/2
  Sum1/1 -> Math Function1/1
  Math Function1/1 -> y/1

== system neuronchainv3/Hebbcon3p2/ /f(ui) ==
  x : Inport
  Constant : Constant  Value=offset
  Constant1 : Constant  Value=slope
  Constant2 : Constant
  Gain : Gain  Gain=-1  SaturateOnIntegerOverflow=on  OutDataTypeStr=Inherit: Same as input  ParamDataTypeStr=Inherit: Same as input
  Math Function : Math  SaturateOnIntegerOverflow=on
  Math Function1 : Math  Operator=reciprocal  SaturateOnIntegerOverflow=on
  Model Info : simulink/Model-Wide Utilities/Model Info  SystemSampleTime=-1  InitialBlockCM=None  BlockCM=None  Frame=on  DisplayStringWithTags=|  HorizontalTextAlignment=Center  LeftAlignmentValue=0.5  SourceBlockDiagram=neuronchainv3  TagMaxNumber=20
      | Model Info
      | %<Creator> Han, Cheol
  Product : Product  SaturateOnIntegerOverflow=on  OutDataTypeStr=Inherit: Same as first input
  Sum : Sum  Inputs=+-  SaturateOnIntegerOverflow=on
  Sum1 : Sum  SaturateOnIntegerOverflow=on
  y : Outport  InitialOutput=0
  wires:
  x/1 -> Sum/1
  Constant/1 -> Sum/2
  Sum/1 -> Product/1
  Constant1/1 -> Product/2
  Product/1 -> Gain/1
  Gain/1 -> Math Function/1
  Math Function/1 -> Sum1/1
  Constant2/1 -> Sum1/2
  Sum1/1 -> Math Function1/1
  Math Function1/1 -> y/1

== system neuronchainv3/Hebbcon3p2/ /f(uj) ==
  x : Inport
  Constant : Constant  Value=offset
  Constant1 : Constant  Value=slope
  Constant2 : Constant
  Gain : Gain  Gain=-1  SaturateOnIntegerOverflow=on  OutDataTypeStr=Inherit: Same as input  ParamDataTypeStr=Inherit: Same as input
  Math Function : Math  SaturateOnIntegerOverflow=on
  Math Function1 : Math  Operator=reciprocal  SaturateOnIntegerOverflow=on
  Model Info : simulink/Model-Wide Utilities/Model Info  SystemSampleTime=-1  InitialBlockCM=None  BlockCM=None  Frame=on  DisplayStringWithTags=|  HorizontalTextAlignment=Center  LeftAlignmentValue=0.5  SourceBlockDiagram=excneuronv3  TagMaxNumber=20
      | Model Info
      | %<Creator> Han, Cheol
  Product : Product  SaturateOnIntegerOverflow=on  OutDataTypeStr=Inherit: Same as first input
  Sum : Sum  Inputs=+-  SaturateOnIntegerOverflow=on
  Sum1 : Sum  SaturateOnIntegerOverflow=on
  y : Outport  InitialOutput=0
  wires:
  x/1 -> Sum/1
  Constant/1 -> Sum/2
  Sum/1 -> Product/1
  Constant1/1 -> Product/2
  Product/1 -> Gain/1
  Gain/1 -> Math Function/1
  Math Function/1 -> Sum1/1
  Constant2/1 -> Sum1/2
  Sum1/1 -> Math Function1/1
  Math Function1/1 -> y/1

== system neuronchainv3/Hebbcon3p2/ /h(ui) ==
  x : Inport
  Constant : Constant  Value=offset
  Constant1 : Constant  Value=slope
  Constant2 : Constant
  Gain : Gain  Gain=-1  SaturateOnIntegerOverflow=on  OutDataTypeStr=Inherit: Same as input  ParamDataTypeStr=Inherit: Same as input
  Math Function : Math  SaturateOnIntegerOverflow=on
  Math Function1 : Math  Operator=reciprocal  SaturateOnIntegerOverflow=on
  Model Info : simulink/Model-Wide Utilities/Model Info  SystemSampleTime=-1  InitialBlockCM=None  BlockCM=None  Frame=on  DisplayStringWithTags=|  HorizontalTextAlignment=Center  LeftAlignmentValue=0.5  SourceBlockDiagram=excneuronv3  TagMaxNumber=20
      | Model Info
      | %<Creator> Han, Cheol
  Product : Product  SaturateOnIntegerOverflow=on  OutDataTypeStr=Inherit: Same as first input
  Sum : Sum  Inputs=+-  SaturateOnIntegerOverflow=on
  Sum1 : Sum  SaturateOnIntegerOverflow=on
  y : Outport  InitialOutput=0
  wires:
  x/1 -> Sum/1
  Constant/1 -> Sum/2
  Sum/1 -> Product/1
  Constant1/1 -> Product/2
  Product/1 -> Gain/1
  Gain/1 -> Math Function/1
  Math Function/1 -> Sum1/1
  Constant2/1 -> Sum1/2
  Sum1/1 -> Math Function1/1
  Math Function1/1 -> y/1

== system neuronchainv3/Hebbcon3p2/ 2/f(ui) ==
  x : Inport
  Constant : Constant  Value=offset
  Constant1 : Constant  Value=slope
  Constant2 : Constant
  Gain : Gain  Gain=-1  SaturateOnIntegerOverflow=on  OutDataTypeStr=Inherit: Same as input  ParamDataTypeStr=Inherit: Same as input
  Math Function : Math  SaturateOnIntegerOverflow=on
  Math Function1 : Math  Operator=reciprocal  SaturateOnIntegerOverflow=on
  Model Info : simulink/Model-Wide Utilities/Model Info  SystemSampleTime=-1  InitialBlockCM=None  BlockCM=None  Frame=on  DisplayStringWithTags=|  HorizontalTextAlignment=Center  LeftAlignmentValue=0.5  SourceBlockDiagram=excneuronv3  TagMaxNumber=20
      | Model Info
      | %<Creator> Han, Cheol
  Product : Product  SaturateOnIntegerOverflow=on  OutDataTypeStr=Inherit: Same as first input
  Sum : Sum  Inputs=+-  SaturateOnIntegerOverflow=on
  Sum1 : Sum  SaturateOnIntegerOverflow=on
  y : Outport  InitialOutput=0
  wires:
  x/1 -> Sum/1
  Constant/1 -> Sum/2
  Sum/1 -> Product/1
  Constant1/1 -> Product/2
  Product/1 -> Gain/1
  Gain/1 -> Math Function/1
  Math Function/1 -> Sum1/1
  Constant2/1 -> Sum1/2
  Sum1/1 -> Math Function1/1
  Math Function1/1 -> y/1

== system neuronchainv3/Hebbcon3p2/ 2/f(uj) ==
  x : Inport
  Constant : Constant  Value=offset
  Constant1 : Constant  Value=slope
  Constant2 : Constant
  Gain : Gain  Gain=-1  SaturateOnIntegerOverflow=on  OutDataTypeStr=Inherit: Same as input  ParamDataTypeStr=Inherit: Same as input
  Math Function : Math  SaturateOnIntegerOverflow=on
  Math Function1 : Math  Operator=reciprocal  SaturateOnIntegerOverflow=on
  Model Info : simulink/Model-Wide Utilities/Model Info  SystemSampleTime=-1  InitialBlockCM=None  BlockCM=None  Frame=on  DisplayStringWithTags=|  HorizontalTextAlignment=Center  LeftAlignmentValue=0.5  SourceBlockDiagram=excneuronv3  TagMaxNumber=20
      | Model Info
      | %<Creator> Han, Cheol
  Product : Product  SaturateOnIntegerOverflow=on  OutDataTypeStr=Inherit: Same as first input
  Sum : Sum  Inputs=+-  SaturateOnIntegerOverflow=on
  Sum1 : Sum  SaturateOnIntegerOverflow=on
  y : Outport  InitialOutput=0
  wires:
  x/1 -> Sum/1
  Constant/1 -> Sum/2
  Sum/1 -> Product/1
  Constant1/1 -> Product/2
  Product/1 -> Gain/1
  Gain/1 -> Math Function/1
  Math Function/1 -> Sum1/1
  Constant2/1 -> Sum1/2
  Sum1/1 -> Math Function1/1
  Math Function1/1 -> y/1

== system neuronchainv3/Hebbcon3p2/ 2/h(ui) ==
  x : Inport
  Constant : Constant  Value=offset
  Constant1 : Constant  Value=slope
  Constant2 : Constant
  Gain : Gain  Gain=-1  SaturateOnIntegerOverflow=on  OutDataTypeStr=Inherit: Same as input  ParamDataTypeStr=Inherit: Same as input
  Math Function : Math  SaturateOnIntegerOverflow=on
  Math Function1 : Math  Operator=reciprocal  SaturateOnIntegerOverflow=on
  Model Info : simulink/Model-Wide Utilities/Model Info  SystemSampleTime=-1  InitialBlockCM=None  BlockCM=None  Frame=on  DisplayStringWithTags=|  HorizontalTextAlignment=Center  LeftAlignmentValue=0.5  SourceBlockDiagram=excneuronv3  TagMaxNumber=20
      | Model Info
      | %<Creator> Han, Cheol
  Product : Product  SaturateOnIntegerOverflow=on  OutDataTypeStr=Inherit: Same as first input
  Sum : Sum  Inputs=+-  SaturateOnIntegerOverflow=on
  Sum1 : Sum  SaturateOnIntegerOverflow=on
  y : Outport  InitialOutput=0
  wires:
  x/1 -> Sum/1
  Constant/1 -> Sum/2
  Sum/1 -> Product/1
  Constant1/1 -> Product/2
  Product/1 -> Gain/1
  Gain/1 -> Math Function/1
  Math Function/1 -> Sum1/1
  Constant2/1 -> Sum1/2
  Sum1/1 -> Math Function1/1
  Math Function1/1 -> y/1

== system neuronchainv3/Hebbcon3p2/11/f(ui) ==
  x : Inport
  Constant : Constant  Value=offset
  Constant1 : Constant  Value=slope
  Constant2 : Constant
  Gain : Gain  Gain=-1  SaturateOnIntegerOverflow=on  OutDataTypeStr=Inherit: Same as input  ParamDataTypeStr=Inherit: Same as input
  Math Function : Math  SaturateOnIntegerOverflow=on
  Math Function1 : Math  Operator=reciprocal  SaturateOnIntegerOverflow=on
  Model Info : simulink/Model-Wide Utilities/Model Info  SystemSampleTime=-1  InitialBlockCM=None  BlockCM=None  Frame=on  DisplayStringWithTags=|  HorizontalTextAlignment=Center  LeftAlignmentValue=0.5  SourceBlockDiagram=excneuronv3  TagMaxNumber=20
      | Model Info
      | %<Creator> Han, Cheol
  Product : Product  SaturateOnIntegerOverflow=on  OutDataTypeStr=Inherit: Same as first input
  Sum : Sum  Inputs=+-  SaturateOnIntegerOverflow=on
  Sum1 : Sum  SaturateOnIntegerOverflow=on
  y : Outport  InitialOutput=0
  wires:
  x/1 -> Sum/1
  Constant/1 -> Sum/2
  Sum/1 -> Product/1
  Constant1/1 -> Product/2
  Product/1 -> Gain/1
  Gain/1 -> Math Function/1
  Math Function/1 -> Sum1/1
  Constant2/1 -> Sum1/2
  Sum1/1 -> Math Function1/1
  Math Function1/1 -> y/1

== system neuronchainv3/Hebbcon3p2/11/f(uj) ==
  x : Inport
  Constant : Constant  Value=offset
  Constant1 : Constant  Value=slope
  Constant2 : Constant
  Gain : Gain  Gain=-1  SaturateOnIntegerOverflow=on  OutDataTypeStr=Inherit: Same as input  ParamDataTypeStr=Inherit: Same as input
  Math Function : Math  SaturateOnIntegerOverflow=on
  Math Function1 : Math  Operator=reciprocal  SaturateOnIntegerOverflow=on
  Model Info : simulink/Model-Wide Utilities/Model Info  SystemSampleTime=-1  InitialBlockCM=None  BlockCM=None  Frame=on  DisplayStringWithTags=|  HorizontalTextAlignment=Center  LeftAlignmentValue=0.5  SourceBlockDiagram=excneuronv3  TagMaxNumber=20
      | Model Info
      | %<Creator> Han, Cheol
  Product : Product  SaturateOnIntegerOverflow=on  OutDataTypeStr=Inherit: Same as first input
  Sum : Sum  Inputs=+-  SaturateOnIntegerOverflow=on
  Sum1 : Sum  SaturateOnIntegerOverflow=on
  y : Outport  InitialOutput=0
  wires:
  x/1 -> Sum/1
  Constant/1 -> Sum/2
  Sum/1 -> Product/1
  Constant1/1 -> Product/2
  Product/1 -> Gain/1
  Gain/1 -> Math Function/1
  Math Function/1 -> Sum1/1
  Constant2/1 -> Sum1/2
  Sum1/1 -> Math Function1/1
  Math Function1/1 -> y/1

== system neuronchainv3/Hebbcon3p2/11/h(ui) ==
  x : Inport
  Constant : Constant  Value=offset
  Constant1 : Constant  Value=slope
  Constant2 : Constant
  Gain : Gain  Gain=-1  SaturateOnIntegerOverflow=on  OutDataTypeStr=Inherit: Same as input  ParamDataTypeStr=Inherit: Same as input
  Math Function : Math  SaturateOnIntegerOverflow=on
  Math Function1 : Math  Operator=reciprocal  SaturateOnIntegerOverflow=on
  Model Info : simulink/Model-Wide Utilities/Model Info  SystemSampleTime=-1  InitialBlockCM=None  BlockCM=None  Frame=on  DisplayStringWithTags=|  HorizontalTextAlignment=Center  LeftAlignmentValue=0.5  SourceBlockDiagram=excneuronv3  TagMaxNumber=20
      | Model Info
      | %<Creator> Han, Cheol
  Product : Product  SaturateOnIntegerOverflow=on  OutDataTypeStr=Inherit: Same as first input
  Sum : Sum  Inputs=+-  SaturateOnIntegerOverflow=on
  Sum1 : Sum  SaturateOnIntegerOverflow=on
  y : Outport  InitialOutput=0
  wires:
  x/1 -> Sum/1
  Constant/1 -> Sum/2
  Sum/1 -> Product/1
  Constant1/1 -> Product/2
  Product/1 -> Gain/1
  Gain/1 -> Math Function/1
  Math Function/1 -> Sum1/1
  Constant2/1 -> Sum1/2
  Sum1/1 -> Math Function1/1
  Math Function1/1 -> y/1

== system neuronchainv3/Hebbcon3p2/12/f(ui) ==
  x : Inport
  Constant : Constant  Value=offset
  Constant1 : Constant  Value=slope
  Constant2 : Constant
  Gain : Gain  Gain=-1  SaturateOnIntegerOverflow=on  OutDataTypeStr=Inherit: Same as input  ParamDataTypeStr=Inherit: Same as input
  Math Function : Math  SaturateOnIntegerOverflow=on
  Math Function1 : Math  Operator=reciprocal  SaturateOnIntegerOverflow=on
  Model Info : simulink/Model-Wide Utilities/Model Info  SystemSampleTime=-1  InitialBlockCM=None  BlockCM=None  Frame=on  DisplayStringWithTags=|  HorizontalTextAlignment=Center  LeftAlignmentValue=0.5  SourceBlockDiagram=excneuronv3  TagMaxNumber=20
      | Model Info
      | %<Creator> Han, Cheol
  Product : Product  SaturateOnIntegerOverflow=on  OutDataTypeStr=Inherit: Same as first input
  Sum : Sum  Inputs=+-  SaturateOnIntegerOverflow=on
  Sum1 : Sum  SaturateOnIntegerOverflow=on
  y : Outport  InitialOutput=0
  wires:
  x/1 -> Sum/1
  Constant/1 -> Sum/2
  Sum/1 -> Product/1
  Constant1/1 -> Product/2
  Product/1 -> Gain/1
  Gain/1 -> Math Function/1
  Math Function/1 -> Sum1/1
  Constant2/1 -> Sum1/2
  Sum1/1 -> Math Function1/1
  Math Function1/1 -> y/1

== system neuronchainv3/Hebbcon3p2/12/f(uj) ==
  x : Inport
  Constant : Constant  Value=offset
  Constant1 : Constant  Value=slope
  Constant2 : Constant
  Gain : Gain  Gain=-1  SaturateOnIntegerOverflow=on  OutDataTypeStr=Inherit: Same as input  ParamDataTypeStr=Inherit: Same as input
  Math Function : Math  SaturateOnIntegerOverflow=on
  Math Function1 : Math  Operator=reciprocal  SaturateOnIntegerOverflow=on
  Model Info : simulink/Model-Wide Utilities/Model Info  SystemSampleTime=-1  InitialBlockCM=None  BlockCM=None  Frame=on  DisplayStringWithTags=|  HorizontalTextAlignment=Center  LeftAlignmentValue=0.5  SourceBlockDiagram=excneuronv3  TagMaxNumber=20
      | Model Info
      | %<Creator> Han, Cheol
  Product : Product  SaturateOnIntegerOverflow=on  OutDataTypeStr=Inherit: Same as first input
  Sum : Sum  Inputs=+-  SaturateOnIntegerOverflow=on
  Sum1 : Sum  SaturateOnIntegerOverflow=on
  y : Outport  InitialOutput=0
  wires:
  x/1 -> Sum/1
  Constant/1 -> Sum/2
  Sum/1 -> Product/1
  Constant1/1 -> Product/2
  Product/1 -> Gain/1
  Gain/1 -> Math Function/1
  Math Function/1 -> Sum1/1
  Constant2/1 -> Sum1/2
  Sum1/1 -> Math Function1/1
  Math Function1/1 -> y/1
